simulink model "Aplicacion"  (R2018a)
settings: Solver=ode45  StartTime=0.0  StopTime=10  RelTol=1e-3  AbsTol=1e-6
undefined symbols (not defined in the file or in its folder): sfunxy2
libraries: neural x1
settings Model: ExtModeTrigMode=oneshot  ExtModeArmWhenConnect=off  TunableVars=prueba  TunableVarsStorageClass=Auto  Creator=matthew  LastModifiedBy=daniel
settings SolverCC: AutoScaleAbsTol=off
settings DataIOCC: SaveFormat=Array  SignalLoggingSaveFormat=ModelDataLogs  SaveOutput=off  SignalLoggingName=sigsOut
settings OptimizationCC: BooleanDataType=off  InitFltsAndDblsToZero=on  LifeSpan=inf
settings DebuggingCC: SaveWithParameterizedLinksMsg=none  UnderspecifiedInitializationDetection=Classic  MergeDetectMultiDrivingBlocksExec=none  SignalResolutionControl=TryResolveAllWithWarning  MultiTaskDSMMsg=warning  MultiTaskCondExecSysMsg=none  SFUnexpectedBacktrackingDiag=warning  SFNoUnconditionalDefaultTransitionDiag=warning  SFExecutionAtInitializationDiag=none
settings HardwareCC: ProdBitPerPointer=32  ProdBitPerSizeT=32  ProdBitPerPtrDiffT=32  ProdLargestAtomicFloat=None  ProdIntDivRoundTo=Undefined  ProdEndianess=Unspecified  ProdWordSize=32  ProdHWDeviceType=32-bit Generic  TargetUnknown=on
settings ModelReferenceCC: PropagateSignalLabelsOutOfModel=off
settings RTWCC: TemplateMakefile=grt_vc.tmf
settings CodeAppCC: StateflowObjectComments=on
settings GRTTargetCC: TargetFcnLib=ansi_tfl_tmw.mat  TargetLangStandard=C89/C90 (ANSI)  CombineOutputUpdateFcns=off  GRTInterface=on
settings ConfigComp: CovMetricSettings=dw  CovHtmlReporting=on  CovSaveCumulativeToWorkspaceVar=on  CovSaveSingleToWorkspaceVar=on  CovExternalEMLEnable=off

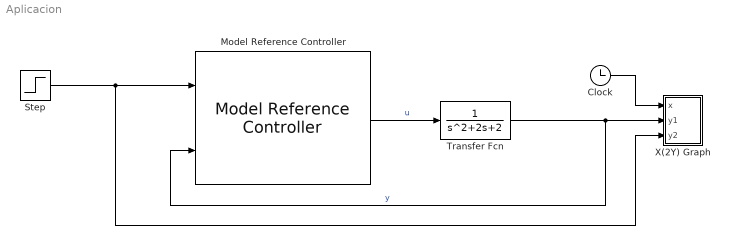
== system Aplicacion ==
  Clock : Clock
  Model Reference Controller : neural/Control Systems/Model Reference Controller  Nrc=2  Nic=2  Njc=2  IW_y=[0.66368920958345822836 -0.58175852157383500796;1.8934721612319460604 1.3048605384932201456;-0.084608480109482228637 -0.53004788008401537702;-0.21991834120073036618 -0.65467857971679677132]  IW_u=[0.11317133838917092792 -0.61323280275157765473;2.1230036700250738413 2.7478046996569438498;0.049650470577029474917 0.56820450270370437273;0.096644251433725902878 -0.061041269640582478118]  IW_r=[0.32977042645063631143 1.5278685087699670486;0.40432994759559831577 -0.58427815160489937618;-0.71821878070901656876 -0.27117951572185938769;0.32295694839951444299 0.007937660872922878974]  B1_c=[-0.29239485258402114765;0.50462369755366054402;-3.4854547349967930359;-3.2590579171615363663]  B2_c=0.76236649018340107986  LW_c=[1.4571517838302792125 -1.3068097654495463011 -2.1376912604158588849 0.42840310779271301156]  retraining_c=2  max_i_int=10  min_i_int=1  max_r_int=10  min_r_int=1  Ts=0.05  S1=5  Ni=2  Nj=2  sim_file=ModeloPlanta  trainfun=trainlm  Use_validation=0  Use_Testing=0  Use_Inc_training=0  Use_previous_weights=1  max_i=4  min_i=0  max_r=2  min_r=0  sam_training=800  sam_training_c=800  epochs=300  epochs_c=20  minp=0.43107606097497219722  maxp=3.9306535988878010812  mint=0  maxt=3.9306535988878010812  Normalize=0  IW=[-0.00046481370185044230308 -0.00038700969444968179485;0.00020777398220152718737 0.00020256950517071164986;0.96007369544888609969 -1.3630238490077795088;-0.026575697535473865457 -0.70457224591983036444;0.36098022257806577917 0.68566508616729981984]  LW1_2=[-0.67568466114499481368 0.3228194084528314689;0.32885817965521785267 -0.15648862510769737111;-0.79632037189371307484 1.2370475995562035809;-0.35992202513773191574 1.4017567517475821859;1.2652548549611446482 -1.4757387207331233991]  LW2_1=[-1.2072580803604306965 5.3669365735436063147 -2.1065007982362460922e-05 -0.00011600349601164302075 -0.00036470742306206750498]  B1=[-0.59696195622506376122;-0.55425436902565616837;-1.2522790536937968842;-1.5287983956842532418;1.058757074583167368]  B2=2.0578642828636146689  S1c=4  Limit_output=0  min_output=-Inf  max_output=Inf  Ref_file=ModeloPlantaReferencia
      settings: SourceProductName=Neural Network Toolbox  SourceProductBaseCode=NN
  Step : Step  Time=0  SampleTime=0
  Transfer Fcn : TransferFcn  Denominator=[1 2 2]
  X(2Y) Graph : Subsystem  LoadFcn=sfunxy2([],[],[],'LoadBlock')  StartFcn=sfunxy2([],[],[],'Start')  StopFcn=sfunxy2([],[],[],'Stop')  mask(X(2Y) scope.){xmin=0, xmax=10, ymin=0, ymax=2, st=-1}
      mask prompts: xmin "x-min:"; xmax "x-max:"; ymin "y-min:"; ymax "y-max:"; st "Sample time:"
      mask help: X(2Y) scope using MATLAB graph window. First input is used as time base. Enter plotting ranges.
      settings: CopyFcn=sfunxy2([],[],[],'CopyBlock')  DeleteFcn=sfunxy2([],[],[],'DeleteBlock')  NameChangeFcn=sfunxy2([],[],[],'NameChange')
      mask Help: This block can be used to explore limit cycles. Look at the m-file sfunxy.m to see how it works.
      mask Display: plot([.05 .95 .95 .05 .05],[.45 .45 .95 .95 .45], 0.5+cos(0:0.1:2*pi)*0.3,0.7+sin(0:0.1:2*pi)*0.2)
  wires:
  Transfer Fcn/1 -> X(2Y) Graph/2(y1), Model Reference Controller/2  "y"
  Model Reference Controller/1 -> Transfer Fcn/1  "u"
  Clock/1 -> X(2Y) Graph/1(x)
  Step/1 -> X(2Y) Graph/3(y2), Model Reference Controller/1

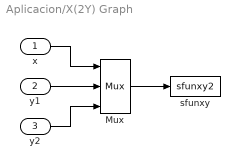
== system Aplicacion/X(2Y) Graph ==
  x : Inport
  y1 : Inport  Port=2
  y2 : Inport  Port=3
  Mux : Mux  Inputs=3
  sfunxy : S-Function  FunctionName=sfunxy2  Parameters=[xmin xmax ymin ymax], st  SFunctionDeploymentMode=off  EnableBusSupport=off
  wires:
  y2/1 -> Mux/3
  y1/1 -> Mux/2
  x/1 -> Mux/1
  Mux/1 -> sfunxy/1
